simulink model "mpc_prueba_raul"  (R2017a)
settings: Solver=VariableStepAuto  StartTime=0.0  StopTime=1  MaxStep=1e-4  RelTol=1e-3
values from neighbouring files (symbols this model uses):
  A = linsys1.A    [MPC_Calculation.m]
  B = linsys1.B    [MPC_Calculation.m]
  C = linsys1.C    [MPC_Calculation.m]
  D = linsys1.D    [MPC_Calculation.m]
libraries: mpclib x1, powerlib x1
settings Model: Creator=Administrador  LastModifiedBy=erich

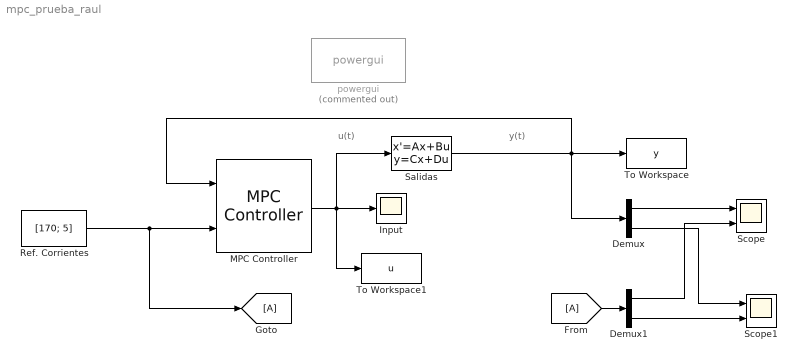
== system mpc_prueba_raul ==
  note: y(t)
  note: u(t)
  Demux : Demux  Outputs=2
  Demux1 : Demux  Outputs=2
  Input : Scope
  MPC Controller : mpclib/MPC Controller  mpcobj=mpcobj  x0=[]  is_multiple=0  enable_value=0  return_u0=off  ref_from_ws=off  ref_signal_name=[]  ref_preview=on  md_from_ws=off  md_signal_name=[]  md_preview=on  from_project=off  project_file=MPCtask.mat  md_inport=off  mv_inport=off  cost_outport=off  return_sequence=off  return_qpstatus=off  return_state=off  state_inport=off  lims_inport=off  ywt_inport=off  is_designfromscratch=0  uwt_inport=off  duwt_inport=off  rhoeps_inport=off  uref_inport=off  n_ts=0.001  n_mv=2  n_md=0  n_ud=0  n_mo=2  n_uo=0  BlockDataType=double  SampleTimeInherited=off  switch_inport=off
  Ref. Corrientes : Constant  Value=[170; 5]
  Salidas : StateSpace  A=A  B=B  C=C  D=D  X0=0
  Scope : Scope  NumInputPorts=2
  Scope1 : Scope  NumInputPorts=2
  To Workspace : ToWorkspace  VariableName=y  SampleTime=-1
      settings: MaxDataPoints=Inf
  To Workspace1 : ToWorkspace  VariableName=u  SampleTime=-1
      settings: MaxDataPoints=Inf
  powergui : powerlib/powergui  Commented=on  SimulationMode=Continuous  SampleTime=50e-6  frequency=60  Iterations=50  frequencyindice=0  Pbase=100e6  ErrMax=1e-4  UnitsV=kV  UnitsW=MW  buscounter=0  FunctionMessages=off  echomessages=off  EnableUseOfTLC=off  CurrentSourceSwitches=off  DisableSnubberDevices=off  DisableRonSwitches=off  DisableVfSwitches=off  DisplayEquations=off  SolverType=Tustin/Backward Euler (TBE)  Interpol=off  ExternalGateDelay=off  methode=off  Ts=100  x0status=blocks  SPID=on  SwTol=0  HookPort=off  RestoreLinks=warning  ResistiveCurrentMeasurement=off  Frange=[0:2:500]  Ylog=off  Xlog=on  ShowGrid=off  save=off  variable=ZData  structure=sps1phPWM1_str  ZoomFFT=on  StartTime=0.1-2/60  cycles=2  DisplayStyle=1  fundamental=60  FreqAxis=off  MaxFrequency=5000  frequencyindicesteady=1  RmsSteady=1  display=off
  wires:
  Ref. Corrientes/1 -> [A], MPC Controller/2
  MPC Controller/1 -> Salidas/1, Input/1, To Workspace1/1
  Salidas/1 -> Demux/1, To Workspace/1, MPC Controller/1
  [A] -> Demux1/1
  Demux/1 -> Scope/1
  Demux1/1 -> Scope/2
  Demux/2 -> Scope1/1
  Demux1/2 -> Scope1/2
